simulink model "SinglePhaseHBridge_Unipolar"  (R2019a)
settings: Solver=ode23tb  StartTime=0  StopTime=0.1  MaxStep=1e-06  RelTol=1e-3
undefined symbols (not defined in the file or in its folder): fm, Lload, Vdc
libraries: simulink x1
settings Model: Creator=tiany  LastModifiedBy=tiany

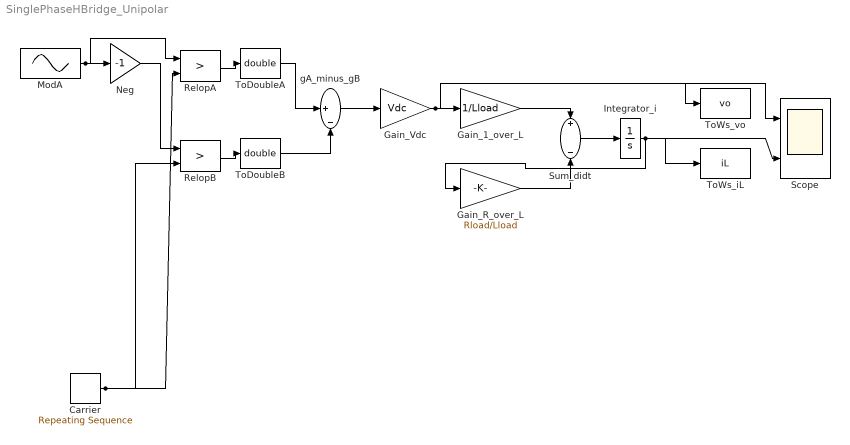
== system SinglePhaseHBridge_Unipolar ==
  Carrier : simulink/Sources/Repeating Sequence  rep_seq_t=[0 2]  rep_seq_y=[0 2]
  Gain_1_over_L : Gain  Gain=1/Lload
  Gain_R_over_L : Gain  Gain=Rload/Lload
  Gain_Vdc : Gain  Gain=Vdc
  Integrator_i : Integrator
  ModA : Sin  Amplitude=0.9  Frequency=2*pi*fm  SampleTime=0
  Neg : Gain  Gain=-1
  RelopA : RelationalOperator  Operator=>  OutDataTypeStr=boolean  RndMeth=Simplest
  RelopB : RelationalOperator  Operator=>  OutDataTypeStr=boolean  RndMeth=Simplest
  Scope : Scope  NumInputPorts=2
  Sum_didt : Sum  Inputs=+-
  ToDoubleA : DataTypeConversion  OutDataTypeStr=double
  ToDoubleB : DataTypeConversion  OutDataTypeStr=double
  ToWs_iL : ToWorkspace  VariableName=iL  SaveFormat=Structure With Time  SampleTime=-1
  ToWs_vo : ToWorkspace  VariableName=vo  SaveFormat=Structure With Time  SampleTime=-1
  gA_minus_gB : Sum  Inputs=|+-
  wires:
  ModA/1 -> Neg/1, RelopA/1
  Carrier/1 -> RelopA/2, RelopB/2
  Neg/1 -> RelopB/1
  RelopA/1 -> ToDoubleA/1
  RelopB/1 -> ToDoubleB/1
  ToDoubleA/1 -> gA_minus_gB/1
  ToDoubleB/1 -> gA_minus_gB/2
  gA_minus_gB/1 -> Gain_Vdc/1
  Gain_Vdc/1 -> Gain_1_over_L/1, Scope/1, ToWs_vo/1
  Gain_1_over_L/1 -> Sum_didt/1
  Integrator_i/1 -> Gain_R_over_L/1, Scope/2, ToWs_iL/1
  Gain_R_over_L/1 -> Sum_didt/2
  Sum_didt/1 -> Integrator_i/1
